simulink model "lab2s"  (R2024b)
settings: Solver=VariableStepAuto  StartTime=0.0  StopTime=10.0  MaxStep=2  RelTol=1e-3
values from neighbouring files (symbols this model uses):
  czas_skok = 1500    [lab2.m]
  dPg = 0.1 * PgN    (= 1000)    [lab2.m]
  k = 3.5 / dPg    (= 0.0035)    [lab2.m]
  T = 3000    [lab2.m]
  Tp0 = (Kp / (Kp + Kd)) * (Pg0 / (K1 + (Kp * Kd) / (Kp + Kd))) + Tzew0    (= 15)    [lab2.m]
settings Model: Creator=Adam  LastModifiedBy=Adam

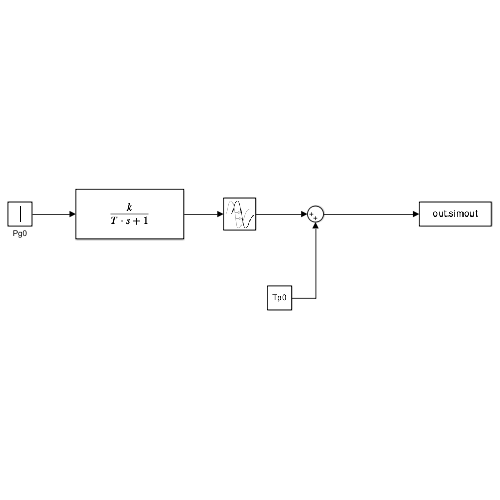
[thumbnail: Simulink's stored preview of the top-level diagram]
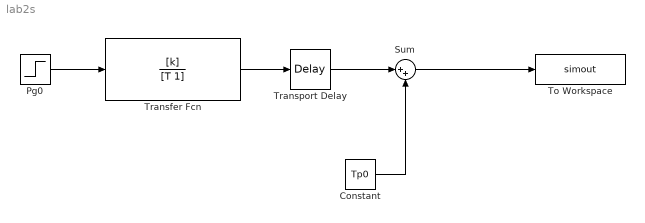
== system lab2s ==
  Constant : Constant  Value=Tp0
  Pg0 : Step  Time=czas_skok  After=dPg  SampleTime=0
  Sum : Sum  Inputs=|++
  To Workspace : ToWorkspace  VariableName=simout  SampleTime=-1
  Transfer Fcn : TransferFcn  Numerator=[k]  Denominator=[T 1]
  Transport Delay : TransportDelay  DelayTime=250
  wires:
  Pg0/1 -> Transfer Fcn/1
  Transfer Fcn/1 -> Transport Delay/1
  Transport Delay/1 -> Sum/1
  Sum/1 -> To Workspace/1
  Constant/1 -> Sum/2
